simulink model "ScalingSignal"  (R2015a)
settings: Solver=ode45  StartTime=0.0  StopTime=10.0  RelTol=1e-3
settings Model: Creator=pc  LastModifiedBy=pc

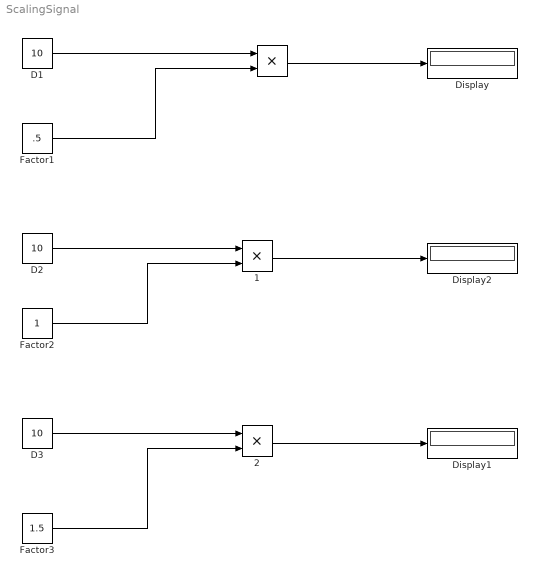
== system ScalingSignal ==
  " " : Product
  " 1" : Product
  " 2" : Product
  D1 : Constant  Value=10
  D2 : Constant  Value=10
  D3 : Constant  Value=10
  Display : Display
  Display1 : Display
  Display2 : Display
  Factor1 : Constant  Value=.5
  Factor2 : Constant
  Factor3 : Constant  Value=1.5
  wires:
  D1/1 -> " "/1
  Factor1/1 -> " "/2
  " "/1 -> Display/1
  " 1"/1 -> Display2/1
  D2/1 -> " 1"/1
  Factor2/1 -> " 1"/2
  D3/1 -> " 2"/1
  Factor3/1 -> " 2"/2
  " 2"/1 -> Display1/1
